simulink model "missile_simulink"  (R2024b)
settings: Solver=VariableStepAuto  StartTime=0.0  StopTime=10.0  RelTol=1e-3
undefined symbols (not defined in the file): A, B, C, D, dT1, dT2, Earth, elev_init, elev_target, K, L, lat_init, lat_obs, lat_target, lon_init, lon_obs, lon_target, Vel, WGS84
libraries: simulink x3, slpidlib x1, aerolibtransform2 x1, aerolibanimutils x1
settings Model: Creator=Harvey  LastModifiedBy=Harvey
settings DebuggingCC: AlgebraicLoopMsg=none

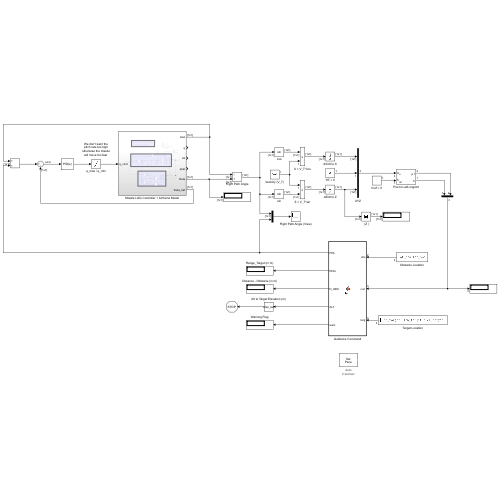
[thumbnail: Simulink's stored preview of the top-level diagram]
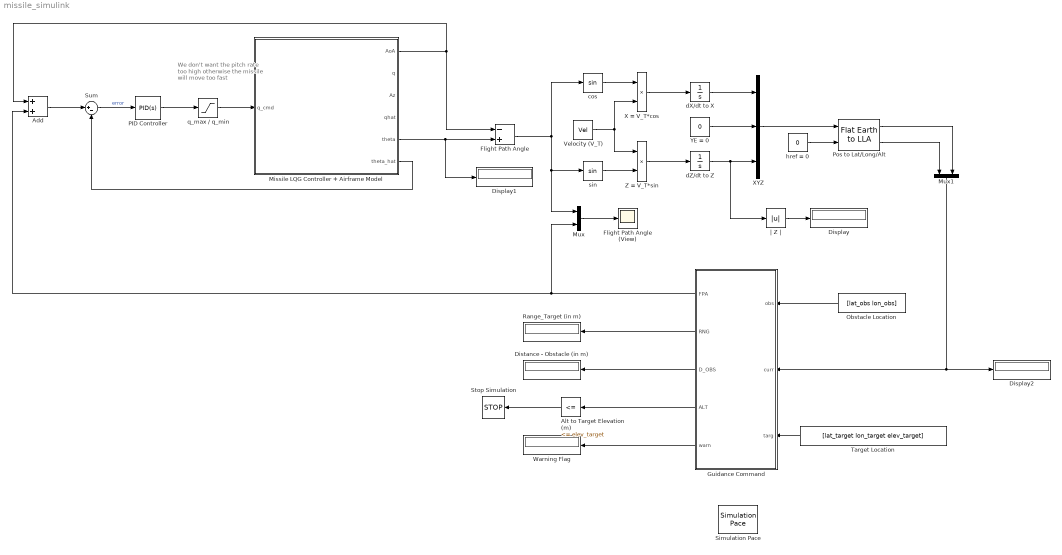
== system missile_simulink ==
  note: We don't want the pitch rate too high otherwise the missile will move too fast
  Add : Sum
  Alt to Target Elevation (m) : simulink/Logic and Bit Operations/Compare To Constant  relop=<=  const=elev_target  OutDataTypeStr=boolean
  Display : Display
  Display1 : Display
  Display2 : Display
  Distance - Obstacle (in m) : Display
  Flight Path Angle : Sum  Inputs=-+
  Flight Path Angle (View) : Scope
  Guidance Command : MATLAB Function  TreatAsAtomicUnit=on
  Missile LQG Controller + Airframe Model : Subsystem
  Mux : Mux  Inputs=2
  Mux1 : Mux  Inputs=2
  Obstacle Location : Constant  Value=[lat_obs lon_obs]
  PID Controller : slpidlib/PID Controller  Controller=PID  Form=Parallel  TimeDomain=Continuous-time  UseExternalTs=off  SampleTime=-1  IntegratorMethod=Forward Euler  FilterMethod=Forward Euler  ControllerParametersSource=internal  P=-1  I=0  UseKiTs=off  D=0  UseExternalDerivativeSource=off  N=100  UseFilter=on  TunerSelectOption=Transfer Function Based (PID Tuner App)  InitialConditionSource=internal  InitialConditionForIntegrator=0  InitialConditionForFilter=0  DifferentiatorICPrevScaledInput=0  ExternalReset=none  TrackingMode=off  Kt=1  LimitOutput=off  SatLimitsSource=internal  UpperSaturationLimit=inf  LowerSaturationLimit=-inf  LinearizeAsGain=on  AntiWindupMode=none  Kb=1  LimitIntegrator=off  UpperIntegratorSaturationLimit=inf  LowerIntegratorSaturationLimit=-inf  POutMin=[]  POutMax=[]  IOutMin=[]  IOutMax=[]  DOutMin=[]  DOutMax=[]  NOutMin=[]  NOutMax=[]  SumOutMin=[]  SumOutMax=[]  SaturationOutMin=[]  SaturationOutMax=[]  PParamMin=[]  PParamMax=[]  IParamMin=[]  IParamMax=[]  DParamMin=[]  DParamMax=[]  NParamMin=[]  NParamMax=[]  KbParamMin=[]  KbParamMax=[]  KtParamMin=[]  KtParamMax=[]  KbOutMin=[]  KbOutMax=[]  KtOutMin=[]  KtOutMax=[]  IntegratorOutMin=[]  IntegratorOutMax=[]  FilterOutMin=[]  FilterOutMax=[]  SumI1OutMin=[]  SumI1OutMax=[]  SumI2OutMin=[]  SumI2OutMax=[]  SumI3OutMin=[]  SumI3OutMax=[]  SumI4OutMin=[]  SumI4OutMax=[]  SumDOutMin=[]  SumDOutMax=[]  DifferentiatorOutMin=[]  DifferentiatorOutMax=[]  FilterDiffOutCoefMin=[]  FilterDiffOutCoefMax=[]  ReciprocalOutMin=[]  ReciprocalOutMax=[]  SumDenOutMin=[]  SumDenOutMax=[]  SumNumOutMin=[]  SumNumOutMax=[]  DivideOutMin=[]  DivideOutMax=[]  UdiffTsProdOutMin=[]  UdiffTsProdOutMax=[]  NTsProdOutMin=[]  NTsProdOutMax=[]  UintegralTsProdOutMin=[]  UintegralTsProdOutMax=[]  UngainTsProdOutMin=[]  UngainTsProdOutMax=[]  ClampingZeroOutDataTypeStr=Inherit: Inherit via back propagation  ClampingZeroOutMin=[]  ClampingZeroOutMax=[]  FilterDenConstantOutDataTypeStr=Inherit: Inherit via back propagation  FilterDenConstantOutMin=[]  FilterDenConstantOutMax=[]  PCopyOutDataTypeStr=Inherit: Inherit via back propagation  PCopyOutMin=[]  PCopyOutMax=[]  NCopyOutDataTypeStr=Inherit: Inherit via back propagation  NCopyOutMin=[]  NCopyOutMax=[]  IntegratorContinuousStateAttributes=''  IntegratorStateMustResolveToSignalObject=off  IntegratorRTWStateStorageClass=Auto  FilterContinuousStateAttributes=''  FilterStateMustResolveToSignalObject=off  FilterRTWStateStorageClass=Auto  ParallelPVariant=InternalParameters  IdealPVariant=Disabled  IVariant=InternalParameters  DVariant=InternalParameters  IntegratorVariant=Continuous  SatVariant=Disabled  AWVariant=Passthrough  PCopyVariant=Disabled  TRVariant=Disabled  FdbkBlocksVariant=Forward  IdealPFdbkVariant=Disabled  SatFdbkVariant=Disabled  DerivativeFilterVariant=ContFilter  NVariant=InternalParameters  NCopyVariant=Disabled  FilterICVariant=InternalICsFilter  IntegratorICVariant=InternalICs  ExternalResetVariant=Disabled  TRSumVariant=Passthrough  SumFdbkVariant=Disabled  SumVariant=Sum_PID  TsampFilterVariant=InternalTs  TsampNgainVariant=Passthrough  TsampIntegralVariant=Disabled_SignalSpec  ExternalSaturationOutDataTypeStr=Inherit: Same as second input  DerivativeSourceVariant=ErrorSignal  PreIntVariant=InternalPreInt
  Pos to Lat/Long/Alt : aerolibtransform2/Flat Earth to LLA  units=Metric (MKS)  ptype=Earth (WGS84)  F=1/298.257223563  R=6378137  refPosPort=off  LL0=[lat_init lon_init]  psi=yaw_init
  Range_Target (in m) : Display
  Simulation Pace : aerolibanimutils/Simulation Pace  SimulationPace=2  SleepMode=Auto  OutputPaceError=off  SampleTime=1/30
  Stop Simulation : Stop
  Sum : Sum  Inputs=|+-
  Target Location : Constant  Value=[lat_target lon_target elev_target]
  Velocity (V_T) : Constant  Value=Vel
  Warning Flag : Display
  X = V_T*cos : Product
  XYZ : Mux  Inputs=3
  YE = 0 : Constant  Value=0
  Z = V_T*sin : Product
  cos : Trigonometry
  dX/dt to X : Integrator
  dZ/dt to Z : Integrator  InitialCondition=-elev_init
  href = 0 : Constant  Value=0
  q_max / q_min : Saturate
  sin : Trigonometry
  | Z | : Abs  SaturateOnIntegerOverflow=off
  wires:
  PID Controller/1 -> q_max / q_min/1
  q_max / q_min/1 -> Missile LQG Controller + Airframe Model/1(q_cmd)
  Sum/1 -> PID Controller/1  "error"
  Add/1 -> Sum/1
  Missile LQG Controller + Airframe Model/6(theta_hat) -> Sum/2
  Missile LQG Controller + Airframe Model/5(theta) -> Display1/1, Flight Path Angle/2
  Missile LQG Controller + Airframe Model/1(AoA) -> Flight Path Angle/1, Add/1
  Flight Path Angle/1 -> cos/1, Mux/1, sin/1
  Mux/1 -> Flight Path Angle (View)/1
  sin/1 -> Z = V_T*sin/2
  cos/1 -> X = V_T*cos/1
  Velocity (V_T)/1 -> Z = V_T*sin/1, X = V_T*cos/2
  X = V_T*cos/1 -> dX/dt to X/1
  Z = V_T*sin/1 -> dZ/dt to Z/1
  YE = 0/1 -> XYZ/2
  dX/dt to X/1 -> XYZ/1
  dZ/dt to Z/1 -> | Z |/1, XYZ/3
  | Z |/1 -> Display/1
  XYZ/1 -> Pos to Lat/Long/Alt/1
  href = 0/1 -> Pos to Lat/Long/Alt/2
  Pos to Lat/Long/Alt/1 -> Mux1/2
  Pos to Lat/Long/Alt/2 -> Mux1/1
  Target Location/1 -> Guidance Command/3(targ)
  Obstacle Location/1 -> Guidance Command/1(obs)
  Mux1/1 -> Display2/1, Guidance Command/2(curr)
  Guidance Command/2(RNG) -> Range_Target (in m)/1
  Guidance Command/3(D_OBS) -> Distance - Obstacle (in m)/1
  Guidance Command/5(warn) -> Warning Flag/1
  Guidance Command/1(FPA) -> Add/2, Mux/2
  Guidance Command/4(ALT) -> Alt to Target Elevation (m)/1
  Alt to Target Elevation (m)/1 -> Stop Simulation/1

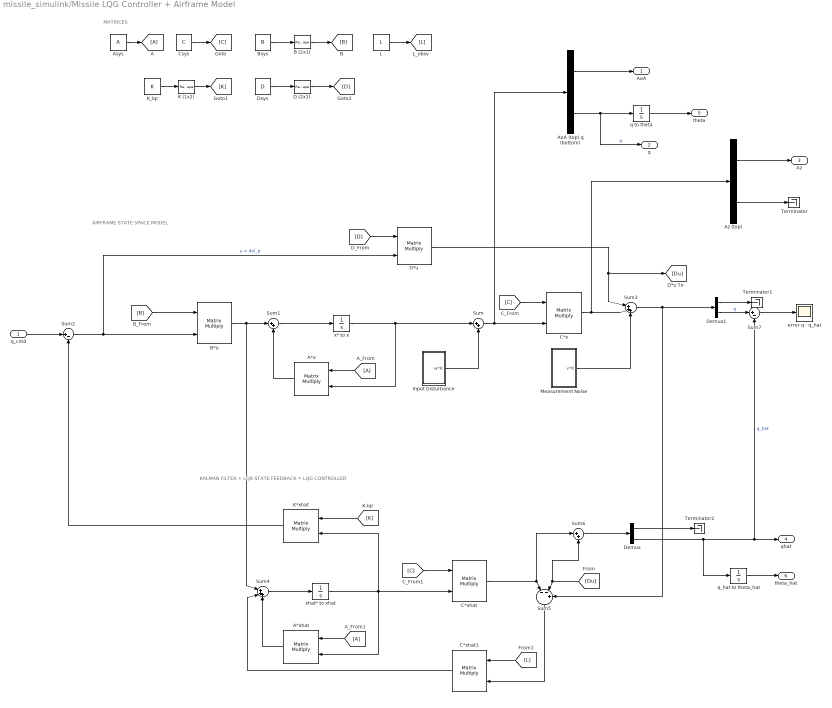
== system missile_simulink/Missile LQG Controller + Airframe Model ==
  note: KALMAN FILTER + LQR STATE FEEDBACK = LQG CONTROLLER
  note: AIRFRAME STATE SPACE MODEL
  note: MATRICES
  q_cmd : Inport
  A : Goto
  A*x : Product  Multiplication=Matrix(*)
  A*xhat : Product  Multiplication=Matrix(*)
  A_From : From
  A_From1 : From
  AoA (top) q (bottom) : Demux  Outputs=2
  Asys : Constant  Value=A
  Az (top) : Demux  Outputs=2
  B (2x1) : Reshape  OutputDimensionality=Customize  OutputDimensions=[2,1]
  B*u : Product  Multiplication=Matrix(*)
  Bsys : Constant  Value=B
  C*x : Product  Multiplication=Matrix(*)
  C*xhat : Product  Multiplication=Matrix(*)
  C*xhat1 : Product  Multiplication=Matrix(*)
  Csys : Constant  Value=C
  D (2x1) : Reshape  OutputDimensionality=Customize  OutputDimensions=[2,1]
  D*u : Product  Multiplication=Matrix(*)
  Demux : Demux  Outputs=2
  Demux1 : Demux  Outputs=2
  Dsys : Constant  Value=D
  Input Disturbance : Subsystem
  K (1x2) : Reshape  OutputDimensionality=Customize  OutputDimensions=[1,2]
  K*xhat : Product  Multiplication=Matrix(*)
  K_lqr : Constant  Value=K
  L : Constant  Value=L
  Measurement Noise : Subsystem
  Sum : Sum  Inputs=|++
  Sum1 : Sum  Inputs=|++
  Sum2 : Sum  Inputs=|+-
  Sum3 : Sum  Inputs=|+++
  Sum4 : Sum  Inputs=|+++
  Sum5 : Sum  Inputs=|--+
  Sum6 : Sum  Inputs=|++
  Sum7 : Sum  Inputs=|+-
  Terminator : Terminator
  Terminator1 : Terminator
  Terminator2 : Terminator
  error q - q_hat : Scope
  q to theta : Integrator
  q_hat to theta_hat : Integrator
  x* to x : Integrator
  xhat* to xhat : Integrator
  AoA : Outport
  q : Outport  Port=2
  Az : Outport  Port=3
  qhat : Outport  Port=4
  theta : Outport  Port=5
  theta_hat : Outport  Port=6
  wires:
  q_hat to theta_hat/1 -> theta_hat/1
  [Du] -> Sum6/2, Sum5/2
  Dsys/1 -> D (2x1)/1
  L/1 -> [L]
  A*xhat/1 -> Sum4/3
  Sum7/1 -> error q - q_hat/1
  A_From/1 -> A*x/1
  C*x/1 -> Az (top)/1, Sum3/2
  Sum6/1 -> Demux/1
  AoA (top) q (bottom)/2 -> q/1, q to theta/1  "q"
  [B] -> B*u/1
  Sum2/1 -> D*u/2, B*u/2  "u = del_p"
  Asys/1 -> A/1
  B*u/1 -> Sum4/1, Sum1/1
  K_lqr/1 -> K (1x2)/1
  Az (top)/1 -> Az/1
  Sum3/1 -> Sum5/3, Demux1/1
  A_From1/1 -> A*xhat/1
  Demux/2 -> q_hat to theta_hat/1, qhat/1, Sum7/2  "q_hat"
  AoA (top) q (bottom)/1 -> AoA/1
  xhat* to xhat/1 -> A*xhat/2, C*xhat/2, K*xhat/2
  Demux1/1 -> Terminator1/1
  B (2x1)/1 -> [B]
  [C] -> C*x/1
  D*u/1 -> [Du], Sum3/1
  K (1x2)/1 -> [K]
  Csys/1 -> [C]
  Sum4/1 -> xhat* to xhat/1
  K*xhat/1 -> Sum2/2
  q to theta/1 -> theta/1
  Demux1/2 -> Sum7/1  "q"
  D (2x1)/1 -> [D]
  C*xhat/1 -> Sum6/1, Sum5/1
  Az (top)/2 -> Terminator/1
  Bsys/1 -> B (2x1)/1
  [D] -> D*u/1
  A*x/1 -> Sum1/2
  x* to x/1 -> A*x/2, Sum/1
  Sum/1 -> AoA (top) q (bottom)/1, C*x/2
  Demux/1 -> Terminator2/1
  Sum1/1 -> x* to x/1
  q_cmd/1 -> Sum2/1
  C*xhat1/1 -> Sum4/2
  [K] -> K*xhat/1
  [L] -> C*xhat1/1
  Sum5/1 -> C*xhat1/2
  [C] -> C*xhat/1
  Input Disturbance/1(w*K) -> Sum/2
  Measurement Noise/1(v*K) -> Sum3/3

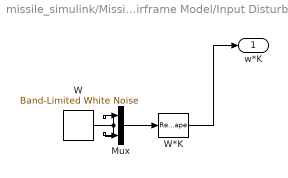
== system missile_simulink/Missile LQG Controller + Airframe Model/Input Disturbance ==
  Mux : Mux  Inputs=2
  W : simulink/Sources/Band-Limited White Noise  Cov=[1e-8]  Ts=dT1  seed=[23341]
  W*K : Reshape  OutputDimensionality=Customize  OutputDimensions=[2,1]
  w*K : Outport
  wires:
  W*K/1 -> w*K/1
  Mux/1 -> W*K/1
  W/1 -> Mux/2, Mux/1

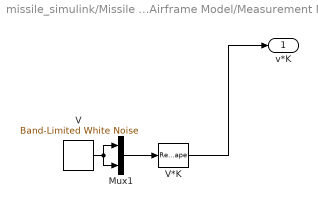
== system missile_simulink/Missile LQG Controller + Airframe Model/Measurement Noise ==
  Mux1 : Mux  Inputs=2
  V : simulink/Sources/Band-Limited White Noise  Cov=[1e-5]  Ts=dT2  seed=[23341]
  V*K : Reshape  OutputDimensionality=Customize  OutputDimensions=[2,1]
  v*K : Outport
  wires:
  V/1 -> Mux1/2, Mux1/1
  Mux1/1 -> V*K/1
  V*K/1 -> v*K/1

== matlab function missile_simulink/Guidance Command ==
  data: obs input; FPA output; curr input; targ input; RNG output; D_OBS output; ALT output; warn output
function [FPA, RNG, D_OBS, ALT, warn] = fcn(obs, curr, targ)

R = 6371e3;
d2r = pi/180;

% Obstacle Location
lat_obs = obs(1);
lon_obs = obs(2);

% Obstacle Threshold (Zone)
thresh = 2e3;

% Target Location
lat_targ = targ(1);
lon_targ = targ(2);
elev_targ = targ(3);

% Current Location
lat_curr = curr(1);
lon_curr = curr(2);
elev_curr = curr(3);

%% Distance To Target
l1 = lat_curr*d2r;
u1 = lon_curr*d2r;
l2 = lat_targ*d2r;
u2 = lon_targ*d2r;
dh = abs(elev_target - elev_curr);

%% Distance From Obstacle
l3 = lat_obs*d2r;
u3 = lon_obs*d2r;

dl = l3 - l1;
du = u3 - u1;

% Haversine Formula
a = sin(dl/2)^2 + cos(l1)*cos(l2)*sin(du/2)^2;
c = 2*atan2(sqrt(a), sqrt(1-a));
d = R*c; % Horizontal Distance (in meters)

%% Current Range (From Target) - range > distance
range = sqrt(d^2 + dh^2);

% Calculate Command Flight Path Setpoint Based on d_obs, range, 
if abs(d_obs)>=thresh
    w = 0;
    fpa_cmd = atan(dh/d);
else
    % When in the obstacle zone, trigger warning
    w = 1;
    fpa_cmd = 0;
end
%% Output Variables

FPA = fpa_cmd;
RNG = range;
D_OBS = d_obs;
ALT = elev_curr;
warn = w;
